simulink model "taller1_uav"  (R2026a)
settings: Solver=ode45  StopTime=t_final
InitFcn:
  | run('/home/sergio/Escritorio/tdc/taller1/init_taller1_simulink.m')
values from neighbouring files (symbols this model uses):
  C_sim = C_full([idx_theta idx_phi idx_p idx_q idx_r], :)    [init_taller1_simulink.m]
  control_mode = 1    [init_taller1_simulink.m]
  D_sim = zeros(5, size(B_full, 2))    [init_taller1_simulink.m]
  dist_amp = cfg.sim.disturbance_amp_rad    [init_taller1_simulink.m]
  dist_freq = 2*pi*cfg.spec.perturbation_hz    [init_taller1_simulink.m]
  noise_sample_time = cfg.sim.dt    [init_taller1_simulink.m]
  noise_var_phi = cfg.spec.noise_power_lat    [init_taller1_simulink.m]
  noise_var_theta = cfg.spec.noise_power_long    [init_taller1_simulink.m]
  t_step = cfg.sim.t_step    [init_taller1_simulink.m]
  umax = cfg.spec.control_limit_rad    [init_taller1_simulink.m]
undefined symbols (not defined in the file or in its folder): A_full, B_full, Kphi_A, Kphi_B, Kphi_C, Kphi_D, Ktheta_A, Ktheta_B, Ktheta_C, Ktheta_D, Kyaw_A, Kyaw_B, Kyaw_C, Kyaw_D, pid_phi_den, pid_phi_num, pid_theta_den, pid_theta_num
settings Model: Creator=sergio  LastModifiedBy=sergio

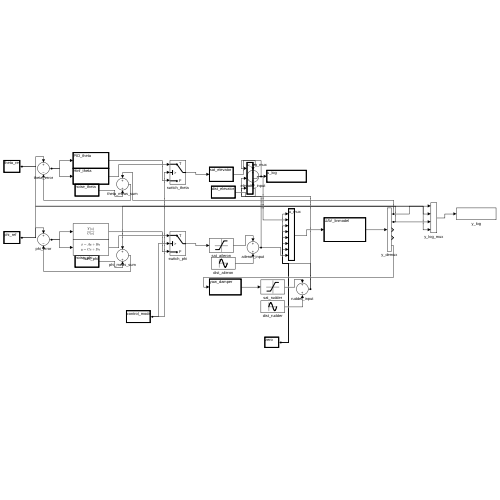
[thumbnail: Simulink's stored preview of the top-level diagram]
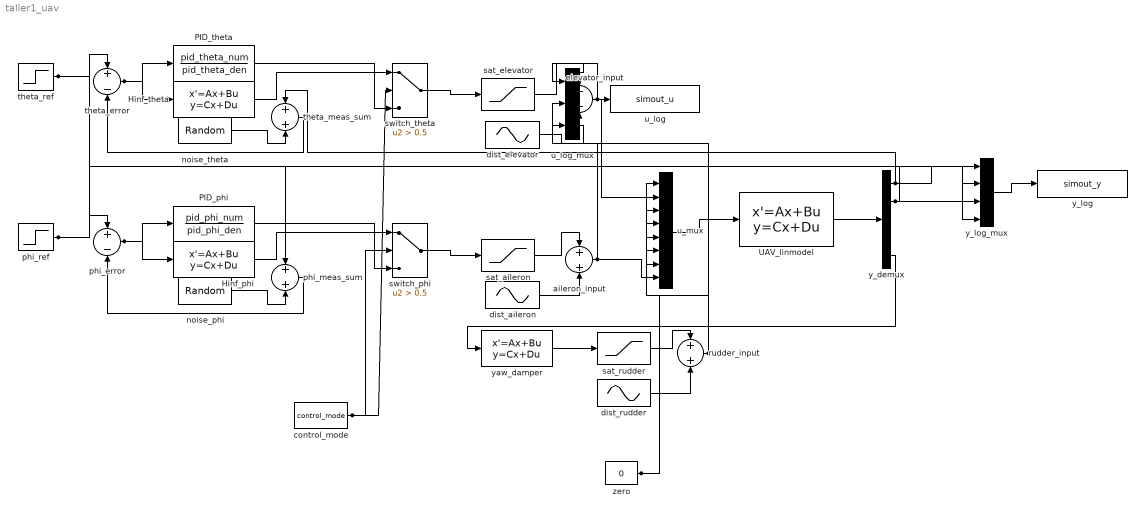
== system taller1_uav ==
  Hinf_phi : StateSpace  A=Kphi_A  B=Kphi_B  C=Kphi_C  D=Kphi_D  InitialCondition=zeros(size(Kphi_A,1),1)
  Hinf_theta : StateSpace  A=Ktheta_A  B=Ktheta_B  C=Ktheta_C  D=Ktheta_D  InitialCondition=zeros(size(Ktheta_A,1),1)
  PID_phi : TransferFcn  Numerator=pid_phi_num  Denominator=pid_phi_den
  PID_theta : TransferFcn  Numerator=pid_theta_num  Denominator=pid_theta_den
  UAV_linmodel : StateSpace  A=A_full  B=B_full  C=C_sim  D=D_sim  InitialCondition=zeros(size(A_full,1),1)
  aileron_input : Sum
  control_mode : Constant  Value=control_mode
  dist_aileron : Sin  Amplitude=dist_amp  Frequency=dist_freq  Phase=pi/4  SampleTime=0
  dist_elevator : Sin  Amplitude=dist_amp  Frequency=dist_freq  SampleTime=0
  dist_rudder : Sin  Amplitude=dist_amp  Frequency=dist_freq  Phase=pi/2  SampleTime=0
  elevator_input : Sum
  noise_phi : RandomNumber  Variance=noise_var_phi  Seed=17  SampleTime=noise_sample_time
  noise_theta : RandomNumber  Variance=noise_var_theta  Seed=11  SampleTime=noise_sample_time
  phi_error : Sum  Inputs=+-
  phi_meas_sum : Sum
  phi_ref : Step  Time=t_step  FinalValue=phi_ref_step  SampleTime=0
  rudder_input : Sum
  sat_aileron : Saturate  UpperLimit=umax  LowerLimit=-umax
  sat_elevator : Saturate  UpperLimit=umax  LowerLimit=-umax
  sat_rudder : Saturate  UpperLimit=umax  LowerLimit=-umax
  switch_phi : Switch  Criteria=u2 > Threshold  Threshold=0.5  SaturateOnIntegerOverflow=off  InputSameDT=off
  switch_theta : Switch  Criteria=u2 > Threshold  Threshold=0.5  SaturateOnIntegerOverflow=off  InputSameDT=off
  theta_error : Sum  Inputs=+-
  theta_meas_sum : Sum
  theta_ref : Step  Time=t_step  FinalValue=theta_ref_step  SampleTime=0
  u_log : ToWorkspace  VariableName=simout_u  SaveFormat=Structure With Time  SampleTime=-1
  u_log_mux : Mux  Inputs=3
  u_mux : Mux  Inputs=8
  y_demux : Demux  Outputs=5
  y_log : ToWorkspace  VariableName=simout_y  SaveFormat=Structure With Time  SampleTime=-1
  y_log_mux : Mux
  yaw_damper : StateSpace  A=Kyaw_A  B=Kyaw_B  C=Kyaw_C  D=Kyaw_D  InitialCondition=0
  zero : Constant  Value=0
  wires:
  UAV_linmodel/1 -> y_demux/1
  u_mux/1 -> UAV_linmodel/1
  y_demux/1 -> theta_meas_sum/1, y_log_mux/1
  noise_theta/1 -> theta_meas_sum/2
  theta_ref/1 -> theta_error/1, y_log_mux/2
  theta_meas_sum/1 -> theta_error/2
  theta_error/1 -> PID_theta/1, Hinf_theta/1
  Hinf_theta/1 -> switch_theta/1
  control_mode/1 -> switch_theta/2, switch_phi/2
  PID_theta/1 -> switch_theta/3
  switch_theta/1 -> sat_elevator/1
  sat_elevator/1 -> elevator_input/1
  dist_elevator/1 -> elevator_input/2
  y_demux/2 -> phi_meas_sum/1, y_log_mux/3
  noise_phi/1 -> phi_meas_sum/2
  phi_ref/1 -> phi_error/1, y_log_mux/4
  phi_meas_sum/1 -> phi_error/2
  phi_error/1 -> PID_phi/1, Hinf_phi/1
  Hinf_phi/1 -> switch_phi/1
  PID_phi/1 -> switch_phi/3
  switch_phi/1 -> sat_aileron/1
  sat_aileron/1 -> aileron_input/1
  dist_aileron/1 -> aileron_input/2
  y_demux/5 -> yaw_damper/1
  yaw_damper/1 -> sat_rudder/1
  sat_rudder/1 -> rudder_input/1
  dist_rudder/1 -> rudder_input/2
  zero/1 -> u_mux/1, u_mux/4, u_mux/5, u_mux/6, u_mux/7
  elevator_input/1 -> u_mux/2, u_log_mux/1
  rudder_input/1 -> u_mux/3, u_log_mux/3
  aileron_input/1 -> u_mux/8, u_log_mux/2
  y_log_mux/1 -> y_log/1
  u_log_mux/1 -> u_log/1
